simulink model "chap4_4sim"  (Simulink 3.00)
settings: Solver=ode45  StartTime=0.0  StopTime=10  RelTol=1e-3
libraries: simulink3 x1
settings Model: LastModifiedBy=liu

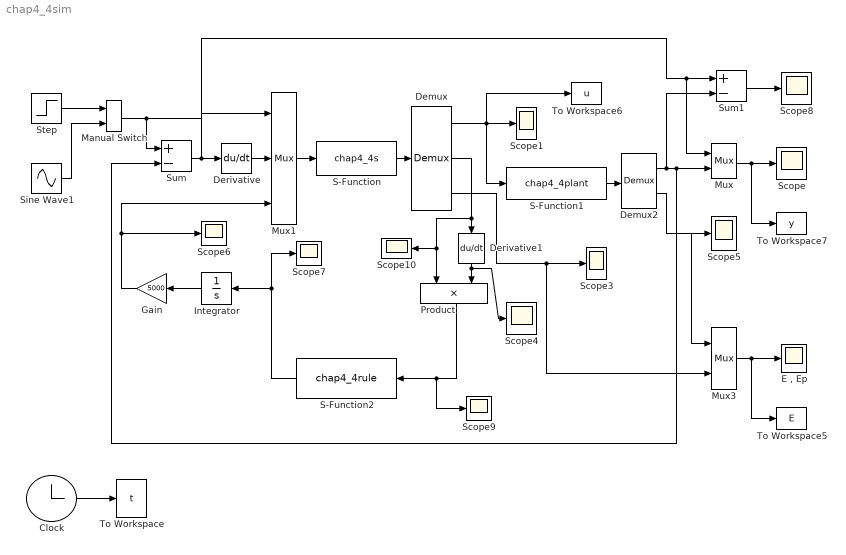
== system chap4_4sim ==
  Clock : Clock
  Demux : Demux  Outputs=3
  Demux2 : Demux  Outputs=2
  Derivative : Derivative
  Derivative1 : Derivative  Orientation=down
  "E , Ep" : Scope
      settings: TimeRange=3  YMin=-225  YMax=225  SaveToWorkspace=off  SaveName=ScopeData  MaxRows=50000
  Gain : Gain  Orientation=left  Gain=5000  SaturateOnIntegerOverflow=on
  Integrator : Integrator  Orientation=left  ExternalReset=none  InitialConditionSource=internal  InitialCondition=0  LimitOutput=off  UpperSaturationLimit=inf  LowerSaturationLimit=-inf  ShowSaturationPort=off  ShowStatePort=off  AbsoluteTolerance=auto
  Manual Switch : simulink3/Nonlinear/Manual Switch  sw=0  action=0
  Mux : Mux  Inputs=2
      settings: DisplayOption=none
  Mux1 : Mux  Inputs=3
      settings: DisplayOption=none
  Mux3 : Mux  Inputs=2
      settings: DisplayOption=none
  Product : Product  Orientation=down  Inputs=2  SaturateOnIntegerOverflow=on
  S-Function : S-Function  FunctionName=chap4_4s  PortCounts=[]  SFunctionModules=''
  S-Function1 : S-Function  FunctionName=chap4_4plant  PortCounts=[]  SFunctionModules=''
  S-Function2 : S-Function  Orientation=left  FunctionName=chap4_4rule  PortCounts=[]  SFunctionModules=''
  Scope{,1,3..10} (10 alike) : Scope
      Scope settings: TimeRange=3  YMin=-1  YMax=1  SaveToWorkspace=off  SaveName=ScopeData  MaxRows=50000
      Scope1 settings: TimeRange=3  YMin=-1.75  YMax=2.25  SaveToWorkspace=off  SaveName=ScopeData  MaxRows=50000
      Scope10 settings: TimeRange=3  YMin=-0.005  YMax=0.065  SaveToWorkspace=off  SaveName=ScopeData  MaxRows=50000
      Scope3 settings: TimeRange=3  YMin=3.25  YMax=9  SaveToWorkspace=off  SaveName=ScopeData
      Scope4 settings: TimeRange=3  YMin=3.25  YMax=9  SaveToWorkspace=off  SaveName=ScopeData
      Scope5 settings: TimeRange=3  YMin=-1  YMax=1  SaveToWorkspace=off  SaveName=ScopeData
      Scope6 settings: TimeRange=1.2  YMin=0.156  YMax=0.165  SaveToWorkspace=off  SaveName=ScopeData  MaxRows=50000
      Scope7 settings: TimeRange=3  YMin=-0.005  YMax=0.065  SaveToWorkspace=off  SaveName=ScopeData  MaxRows=50000
      Scope8 settings: TimeRange=3  YMin=1.475e-005  YMax=2.025e-005  SaveToWorkspace=off  SaveName=ScopeData  MaxRows=50000
      Scope9 settings: TimeRange=3  YMin=-1  YMax=3.5  SaveToWorkspace=off  SaveName=ScopeData  MaxRows=50000
  Sine Wave1 : Sin  Amplitude=1  Frequency=0.5*2*pi  Phase=0  SampleTime=0
  Step : Step  Time=0  Before=0  After=1  SampleTime=0
  Sum : Sum  Inputs=+-  SaturateOnIntegerOverflow=on
  Sum1 : Sum  Inputs=+-  SaturateOnIntegerOverflow=on
  To Workspace : ToWorkspace  VariableName=t  SampleTime=-1  SaveFormat=Matrix
  To Workspace5 : ToWorkspace  VariableName=E  SampleTime=-1  SaveFormat=Matrix
  To Workspace6 : ToWorkspace  VariableName=u  SampleTime=-1  SaveFormat=Matrix
  To Workspace7 : ToWorkspace  VariableName=y  SampleTime=-1  SaveFormat=Matrix
  wires:
  Mux1/1 -> S-Function/1
  Derivative/1 -> Mux1/2
  Sum/1 -> Mux1/1, Derivative/1
  S-Function2/1 -> Scope7/1, Integrator/1
  Gain/1 -> Mux1/3, Scope6/1
  Integrator/1 -> Gain/1
  Step/1 -> Manual Switch/1
  Sine Wave1/1 -> Manual Switch/2
  Manual Switch/1 -> Sum/1, Sum1/1, Mux/1
  S-Function/1 -> Demux/1
  Demux/2 -> Derivative1/1, Product/1, Scope10/1
  Demux/1 -> Scope1/1, To Workspace6/1, S-Function1/1
  S-Function1/1 -> Demux2/1
  Demux2/1 -> Mux/2, Sum/2, Sum1/2
  Sum1/1 -> Scope8/1
  Demux2/2 -> Scope5/1, Mux3/1
  Demux/3 -> Scope3/1, Mux3/2
  Mux3/1 -> "E , Ep"/1, To Workspace5/1
  Mux/1 -> Scope/1, To Workspace7/1
  Product/1 -> S-Function2/1, Scope9/1
  Derivative1/1 -> Product/2, Scope4/1
  Clock/1 -> To Workspace/1
